simulink model "temperature"  (R2024b)
settings: Solver=VariableStepAuto  StartTime=0.0  StopTime=10  RelTol=1e-3
settings Model: Creator=HP  LastModifiedBy=HP

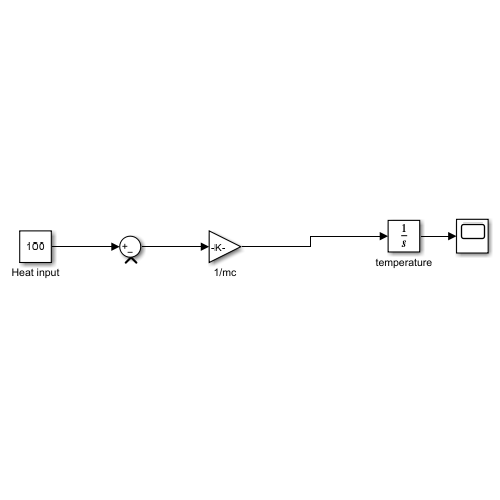
[thumbnail: Simulink's stored preview of the top-level diagram]
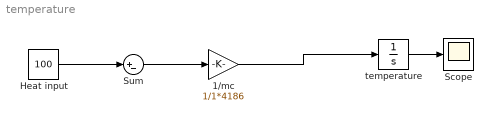
== system temperature ==
  1/mc : Gain  Gain=1/1*4186
  Heat input : Constant  Value=100
  Scope : Scope
  Sum : Sum  Inputs=|+-
  temperature : Integrator  InitialCondition=25
  wires:
  Heat input/1 -> Sum/1
  Sum/1 -> 1/mc/1
  1/mc/1 -> temperature/1
  temperature/1 -> Scope/1
